simulink model "spm_control_sensorless_stc"  (R2021a)
settings: Solver=VariableStepAuto  StartTime=0.0  StopTime=3.0  FixedStep=1e-4  RelTol=1e-5
InitFcn:
  | bldc_data
  | test_data
values from neighbouring files (symbols this model uses):
  b = T_nom/Q_nom    (= 61.8430636014)    [bldc_data.m]
  current_limit = 300    [bldc_data.m]
  flux_obs_gain = 4e4    (= 40000)    [bldc_data.m]
  Jm = 0.3*0.05^2    (= 0.00075)    [bldc_data.m]
  theta_obs_gain = 2e6    (= 2000000)    [bldc_data.m]
undefined symbols (not defined in the file or in its folder): fluid, p, pmsm, r, speed_obs, stc
libraries: mcbcontrolslib x4, pid_lib x3, autolibpmsmexterior x1
settings Model: OrderedModelArguments=off  Creator=Rodrigo  LastModifiedBy=Rodrigo

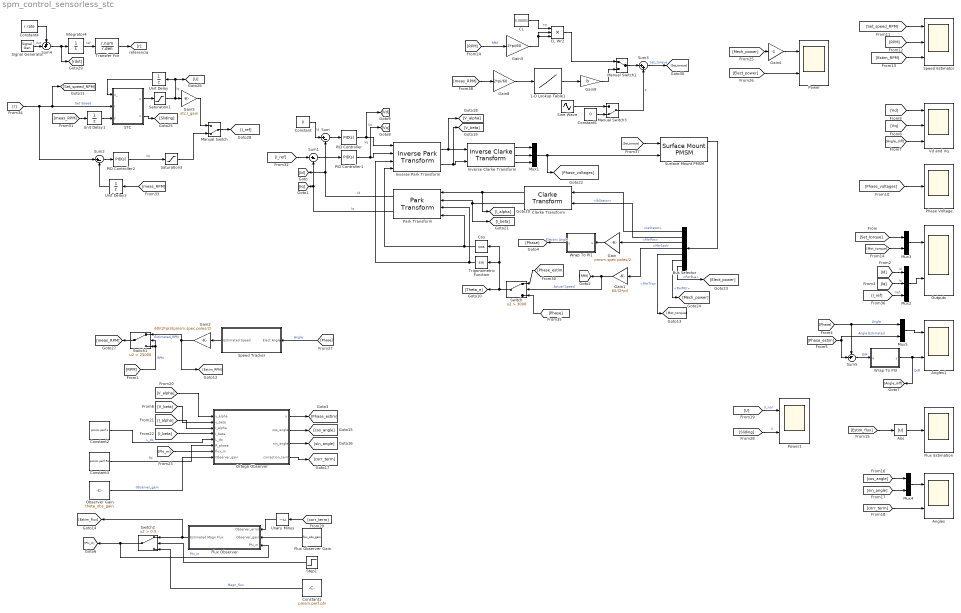
== system spm_control_sensorless_stc ==
  1-D Lookup Table1 : Lookup_n-D  NumberOfTableDimensions=1  BreakpointsForDimension1=fluid.W  Table=fluid.P  InternalRulePriority=Speed  RndMeth=Simplest  InputSameDT=on
  Abs : Abs
  Angles : Scope  NumInputPorts=2
  Angles1 : Scope  NumInputPorts=2
  Bus Selector : BusSelector  OutputSignals=IaStator,IbStator,MtrPos,MtrSpd,MtrTrq,PwrInfo.PwrTrnsfrd.PwrMtr,PwrInfo.PwrTrnsfrd.PwrBus
  CL : Constant  Value=0.00001
  CL Wr2 : Product  Inputs=3
  Clarke Transform : mcbcontrolslib/Clarke Transform  VariantControl=Variant2
  Constant : Constant  Value=0
  Constant1 : Constant  Value=pmsm.perf.phi
  Constant2 : Constant  Value=pmsm.perf.L
  Constant3 : Constant  Value=pmsm.perf.Rs
  Constant4 : Constant  Value=r.rate
  Constant5 : Constant  Value=0
  Cos : Trigonometry  Operator=cos
  Flux Estimation : Scope
  Flux Observer : Subsystem
  Flux Observer Gain : Constant  Value=flux_obs_gain
  Gain : Gain  Gain=pmsm.spec.poles/2
  Gain1 : Gain  Gain=60/(2*pi)
  Gain2 : Gain  Gain=60/(2*pi)/(pmsm.spec.poles/2)
  Gain3 : Gain  Gain=2*pi/60
  Gain4 : Gain  Gain=-1
  Gain5 : Gain  Gain=stc.I_gain
  Gain8 : Gain  Gain=2*pi/60
  Gain9 : Gain  Gain=b
  Integrator4 : Integrator  InitialCondition=r.off  LimitOutput=on  UpperSaturationLimit=r.lim  LowerSaturationLimit=0
  Inverse Clarke Transform : mcbcontrolslib/Inverse Clarke Transform
      settings: SourceProductBaseCode=MT
  Inverse Park Transform : mcbcontrolslib/Inverse Park Transform  AxisAlignment=D-axis
  Manual Switch : ManualSwitch  CurrentSetting=0
  Manual Switch1 : ManualSwitch
  Manual Switch3 : ManualSwitch  CurrentSetting=0
  Mux1 : Mux  Inputs=3
  Mux2 : Mux  Inputs=3
  Mux3 : Mux  Inputs=2
  Mux4 : Mux  Inputs=2
  Mux5 : Mux  Inputs=2
  Observer Gain : Constant  Value=theta_obs_gain
  Ortega Observer : Subsystem
  Outputs : Scope  NumInputPorts=2
  PID Controller : pid_lib/PID Controller  Controller=PID  Form=Parallel  TimeDomain=Continuous-time  UseExternalTs=off  SampleTime=-1  IntegratorMethod=Forward Euler  FilterMethod=Forward Euler  ControllerParametersSource=internal  P=3  I=0.3  D=0.1  UseFilter=on  N=100  TunerSelectOption=Transfer Function Based (PID Tuner App)  InitialConditionSource=internal  InitialConditionForIntegrator=0  InitialConditionForFilter=0  DifferentiatorICPrevScaledInput=0  ExternalReset=none  TrackingMode=off  Kt=1  LimitOutput=off  SatLimitsSource=internal  UpperSaturationLimit=inf  LowerSaturationLimit=-inf  LinearizeAsGain=on  AntiWindupMode=none  Kb=1  POutMin=[]  POutMax=[]  IOutMin=[]  IOutMax=[]  DOutMin=[]  DOutMax=[]  NOutMin=[]  NOutMax=[]  SumOutMin=[]  SumOutMax=[]  SaturationOutMin=[]  SaturationOutMax=[]  PParamMin=[]  PParamMax=[]  IParamMin=[]  IParamMax=[]  DParamMin=[]  DParamMax=[]  NParamMin=[]  NParamMax=[]  KbParamMin=[]  KbParamMax=[]  KtParamMin=[]  KtParamMax=[]  KbOutMin=[]  KbOutMax=[]  KtOutMin=[]  KtOutMax=[]  IntegratorOutMin=[]  IntegratorOutMax=[]  FilterOutMin=[]  FilterOutMax=[]  SumI1OutMin=[]  SumI1OutMax=[]  SumI2OutMin=[]  SumI2OutMax=[]  SumI3OutMin=[]  SumI3OutMax=[]  SumI4OutMin=[]  SumI4OutMax=[]  SumDOutMin=[]  SumDOutMax=[]  DifferentiatorOutMin=[]  DifferentiatorOutMax=[]  FilterDiffOutCoefMin=[]  FilterDiffOutCoefMax=[]  ReciprocalOutMin=[]  ReciprocalOutMax=[]  SumDenOutMin=[]  SumDenOutMax=[]  SumNumOutMin=[]  SumNumOutMax=[]  DivideOutMin=[]  DivideOutMax=[]  UdiffTsProdOutMin=[]  UdiffTsProdOutMax=[]  NTsProdOutMin=[]  NTsProdOutMax=[]  UintegralTsProdOutMin=[]  UintegralTsProdOutMax=[]  UngainTsProdOutMin=[]  UngainTsProdOutMax=[]  IntegratorContinuousStateAttributes=''  IntegratorStateMustResolveToSignalObject=off  IntegratorRTWStateStorageClass=Auto  FilterContinuousStateAttributes=''  FilterStateMustResolveToSignalObject=off  FilterRTWStateStorageClass=Auto  ParallelPVariant=InternalParameters  IdealPVariant=Disabled  IVariant=InternalParameters  DVariant=InternalParameters  IntegratorVariant=Continuous  SatVariant=Disabled  AWVariant=Passthrough  PCopyVariant=Disabled  TRVariant=Disabled  FdbkBlocksVariant=Forward  IdealPFdbkVariant=Disabled  SatFdbkVariant=Disabled  DerivativeFilterVariant=ContFilter  NVariant=InternalParameters  NCopyVariant=Disabled  FilterICVariant=InternalICsFilter  IntegratorICVariant=InternalICs  ExternalResetVariant=Disabled  TRSumVariant=Passthrough  SumFdbkVariant=Disabled  SumVariant=Sum_PID  TsampFilterVariant=InternalTs  TsampNgainVariant=Passthrough  TsampIntegralVariant=Passthrough  ExternalSaturationOutDataTypeStr=Inherit: Same as second input
  PID Controller1 : pid_lib/PID Controller  Controller=PID  Form=Parallel  TimeDomain=Continuous-time  UseExternalTs=off  SampleTime=-1  IntegratorMethod=Forward Euler  FilterMethod=Forward Euler  ControllerParametersSource=internal  P=6  I=2  D=0.3  UseFilter=on  N=100  TunerSelectOption=Transfer Function Based (PID Tuner App)  InitialConditionSource=internal  InitialConditionForIntegrator=0  InitialConditionForFilter=0  DifferentiatorICPrevScaledInput=0  ExternalReset=none  TrackingMode=off  Kt=1  LimitOutput=off  SatLimitsSource=internal  UpperSaturationLimit=inf  LowerSaturationLimit=-inf  LinearizeAsGain=on  AntiWindupMode=none  Kb=1  POutMin=[]  POutMax=[]  IOutMin=[]  IOutMax=[]  DOutMin=[]  DOutMax=[]  NOutMin=[]  NOutMax=[]  SumOutMin=[]  SumOutMax=[]  SaturationOutMin=[]  SaturationOutMax=[]  PParamMin=[]  PParamMax=[]  IParamMin=[]  IParamMax=[]  DParamMin=[]  DParamMax=[]  NParamMin=[]  NParamMax=[]  KbParamMin=[]  KbParamMax=[]  KtParamMin=[]  KtParamMax=[]  KbOutMin=[]  KbOutMax=[]  KtOutMin=[]  KtOutMax=[]  IntegratorOutMin=[]  IntegratorOutMax=[]  FilterOutMin=[]  FilterOutMax=[]  SumI1OutMin=[]  SumI1OutMax=[]  SumI2OutMin=[]  SumI2OutMax=[]  SumI3OutMin=[]  SumI3OutMax=[]  SumI4OutMin=[]  SumI4OutMax=[]  SumDOutMin=[]  SumDOutMax=[]  DifferentiatorOutMin=[]  DifferentiatorOutMax=[]  FilterDiffOutCoefMin=[]  FilterDiffOutCoefMax=[]  ReciprocalOutMin=[]  ReciprocalOutMax=[]  SumDenOutMin=[]  SumDenOutMax=[]  SumNumOutMin=[]  SumNumOutMax=[]  DivideOutMin=[]  DivideOutMax=[]  UdiffTsProdOutMin=[]  UdiffTsProdOutMax=[]  NTsProdOutMin=[]  NTsProdOutMax=[]  UintegralTsProdOutMin=[]  UintegralTsProdOutMax=[]  UngainTsProdOutMin=[]  UngainTsProdOutMax=[]  IntegratorContinuousStateAttributes=''  IntegratorStateMustResolveToSignalObject=off  IntegratorRTWStateStorageClass=Auto  FilterContinuousStateAttributes=''  FilterStateMustResolveToSignalObject=off  FilterRTWStateStorageClass=Auto  ParallelPVariant=InternalParameters  IdealPVariant=Disabled  IVariant=InternalParameters  DVariant=InternalParameters  IntegratorVariant=Continuous  SatVariant=Disabled  AWVariant=Passthrough  PCopyVariant=Disabled  TRVariant=Disabled  FdbkBlocksVariant=Forward  IdealPFdbkVariant=Disabled  SatFdbkVariant=Disabled  DerivativeFilterVariant=ContFilter  NVariant=InternalParameters  NCopyVariant=Disabled  FilterICVariant=InternalICsFilter  IntegratorICVariant=InternalICs  ExternalResetVariant=Disabled  TRSumVariant=Passthrough  SumFdbkVariant=Disabled  SumVariant=Sum_PID  TsampFilterVariant=InternalTs  TsampNgainVariant=Passthrough  TsampIntegralVariant=Passthrough  ExternalSaturationOutDataTypeStr=Inherit: Same as second input
  PID Controller2 : pid_lib/PID Controller  Controller=PID  Form=Parallel  TimeDomain=Continuous-time  UseExternalTs=off  SampleTime=-1  IntegratorMethod=Forward Euler  FilterMethod=Forward Euler  ControllerParametersSource=internal  P=0.009  I=0.06  D=0  UseFilter=on  N=100  TunerSelectOption=Transfer Function Based (PID Tuner App)  InitialConditionSource=internal  InitialConditionForIntegrator=0  InitialConditionForFilter=0  DifferentiatorICPrevScaledInput=0  ExternalReset=none  TrackingMode=off  Kt=1  LimitOutput=off  SatLimitsSource=internal  UpperSaturationLimit=inf  LowerSaturationLimit=-inf  LinearizeAsGain=on  AntiWindupMode=none  Kb=1  POutMin=[]  POutMax=[]  IOutMin=[]  IOutMax=[]  DOutMin=[]  DOutMax=[]  NOutMin=[]  NOutMax=[]  SumOutMin=[]  SumOutMax=[]  SaturationOutMin=[]  SaturationOutMax=[]  PParamMin=[]  PParamMax=[]  IParamMin=[]  IParamMax=[]  DParamMin=[]  DParamMax=[]  NParamMin=[]  NParamMax=[]  KbParamMin=[]  KbParamMax=[]  KtParamMin=[]  KtParamMax=[]  KbOutMin=[]  KbOutMax=[]  KtOutMin=[]  KtOutMax=[]  IntegratorOutMin=[]  IntegratorOutMax=[]  FilterOutMin=[]  FilterOutMax=[]  SumI1OutMin=[]  SumI1OutMax=[]  SumI2OutMin=[]  SumI2OutMax=[]  SumI3OutMin=[]  SumI3OutMax=[]  SumI4OutMin=[]  SumI4OutMax=[]  SumDOutMin=[]  SumDOutMax=[]  DifferentiatorOutMin=[]  DifferentiatorOutMax=[]  FilterDiffOutCoefMin=[]  FilterDiffOutCoefMax=[]  ReciprocalOutMin=[]  ReciprocalOutMax=[]  SumDenOutMin=[]  SumDenOutMax=[]  SumNumOutMin=[]  SumNumOutMax=[]  DivideOutMin=[]  DivideOutMax=[]  UdiffTsProdOutMin=[]  UdiffTsProdOutMax=[]  NTsProdOutMin=[]  NTsProdOutMax=[]  UintegralTsProdOutMin=[]  UintegralTsProdOutMax=[]  UngainTsProdOutMin=[]  UngainTsProdOutMax=[]  IntegratorContinuousStateAttributes=''  IntegratorStateMustResolveToSignalObject=off  IntegratorRTWStateStorageClass=Auto  FilterContinuousStateAttributes=''  FilterStateMustResolveToSignalObject=off  FilterRTWStateStorageClass=Auto  ParallelPVariant=InternalParameters  IdealPVariant=Disabled  IVariant=InternalParameters  DVariant=InternalParameters  IntegratorVariant=Continuous  SatVariant=Disabled  AWVariant=Passthrough  PCopyVariant=Disabled  TRVariant=Disabled  FdbkBlocksVariant=Forward  IdealPFdbkVariant=Disabled  SatFdbkVariant=Disabled  DerivativeFilterVariant=ContFilter  NVariant=InternalParameters  NCopyVariant=Disabled  FilterICVariant=InternalICsFilter  IntegratorICVariant=InternalICs  ExternalResetVariant=Disabled  TRSumVariant=Passthrough  SumFdbkVariant=Disabled  SumVariant=Sum_PID  TsampFilterVariant=InternalTs  TsampNgainVariant=Passthrough  TsampIntegralVariant=Passthrough  ExternalSaturationOutDataTypeStr=Inherit: Same as second input
  Park Transform : mcbcontrolslib/Park Transform  AxisAlignment=D-axis
      settings: SourceProductBaseCode=MT
  Phase Voltage : Scope
  Power : Scope  NumInputPorts=2
  Power1 : Scope  NumInputPorts=2
  STC : MATLAB Function  TreatAsAtomicUnit=on  SystemSampleTime=stc.ts
  Saturation1 : Saturate  UpperLimit=stc.UM  LowerLimit=-stc.UM
  Saturation3 : Saturate  UpperLimit=current_limit  LowerLimit=-current_limit
  Signal Generator : SignalGenerator  Amplitude=r.a  Frequency=r.f
  Sine Wave : Sin  Amplitude=p.a  Frequency=p.w  SampleTime=0
  Speed Estimator : Scope  NumInputPorts=3
  Speed Tracker : Subsystem
  Step1 : Step  Time=0.01  After=2  SampleTime=0
  Sum : Sum  Inputs=|+-
  Sum1 : Sum  Inputs=|+-
  Sum2 : Sum  Inputs=|+-
  Sum3 : Sum  Inputs=|++
  Sum4 : Sum  Inputs=++|
  Sum5 : Sum  Inputs=-+|
  Surface Mount PMSM : autolibpmsmexterior/Surface Mount PMSM  port_config=Torque  sim_type=Continuous  Ts=0.001  P=pmsm.spec.poles/2  Rs=pmsm.perf.Rph  Ldq_=pmsm.perf.L  KConstText=Permanent flux linkage constant (lambda_pm):  lambda_pm=pmsm.perf.phi  Ke=159.9771  Kt=1.323  mechanical=[Jm, 0.0001, 0.2]  idq0=[0 0]  theta_init=0  omega_init=0  KConst=pmsm.perf.phi  lambda_pm_calc=pmsm.perf.phi  RefBlkName='autolibpmsmexterior/Surface Mount PMSM'  aMode=5  Ldq="[0.0017      0.0017]"
      settings: SourceProductBaseCode=PW,DR,MT,UV,VE
  Switch : Switch  Criteria=u2 > Threshold  Threshold=3000
  Switch1 : Switch  Criteria=u2 > Threshold  Threshold=25000
  Switch2 : Switch  Criteria=u2 > Threshold  Threshold=0.5
  Transfer Fcn : TransferFcn  Numerator=r.num  Denominator=r.den
  Trigonometric Function : Trigonometry
  Unary Minus : UnaryMinus
  Unit Delay : UnitDelay  SampleTime=-1  HasFrameUpgradeWarning=on
  Unit Delay1 : UnitDelay  SampleTime=-1  HasFrameUpgradeWarning=on
  Unit Delay2 : UnitDelay  SampleTime=-1  HasFrameUpgradeWarning=on
  Vd and Vq : Scope  NumInputPorts=3
  Wrap To PI1 : MATLAB Function  TreatAsAtomicUnit=on
  Wrap To PI3 : MATLAB Function  TreatAsAtomicUnit=on
  wires:
  Inverse Clarke Transform/1 -> Mux1/1
  Inverse Clarke Transform/2 -> Mux1/2
  Inverse Clarke Transform/3 -> Mux1/3
  Inverse Park Transform/1 -> [V_alpha], Inverse Clarke Transform/1
  Inverse Park Transform/2 -> [V_beta], Inverse Clarke Transform/2
  Clarke Transform/1 -> [I_alpha], Park Transform/1
  Clarke Transform/2 -> [I_beta], Park Transform/2
  PID Controller/1 -> [Vd], Inverse Park Transform/1  "Vd"
  PID Controller1/1 -> [Vq], Inverse Park Transform/2  "Vq"
  Sum/1 -> PID Controller/1
  Sum1/1 -> PID Controller1/1
  Park Transform/1 -> [Id], Sum/2  "Id"
  Park Transform/2 -> [Iq], Sum1/2  "Iq"
  Saturation1/1 -> Gain5/1, [U], Unit Delay/1  "Iq"
  Constant/1 -> Sum/1  "Id"
  Cos/1 -> Park Transform/4, Inverse Park Transform/4
  Trigonometric Function/1 -> Park Transform/3, Inverse Park Transform/3
  Surface Mount PMSM/1 -> Bus Selector/1
  Bus Selector/3 -> Gain/1  "<MtrPos>"
  Bus Selector/1 -> Clarke Transform/1  "<IaStator>"
  Bus Selector/2 -> Clarke Transform/2  "<IbStator>"
  Bus Selector/4 -> Gain1/1  "<MtrSpd>"
  [r] -> Sum2/1, [Set_speed_RPM], STC/2(r)  "Set Speed"
  Speed Tracker/1(Estimated Speed) -> Gain2/1
  Gain/1 -> Wrap To PI1/1(u)
  Wrap To PI1/1(y) -> [Phase]  "Electric Angle"
  Switch/1 -> Cos/1, Trigonometric Function/1, [Theta_e]
  Gain2/1 -> [Estim_RPM], Switch1/1  "Estimated_RPM"
  Gain1/1 -> Switch/2, [RPM]  "Actual Speed"
  [RPM] -> Switch1/2, Switch1/3  "RPM"
  [Set_torque] -> Mux3/1
  [Iq] -> Mux2/2  "Iq"
  [Id] -> Mux2/1  "Id"
  [Phase_estim] -> Sum5/2, Mux5/2  "Angle Estimated"
  [Phase] -> Mux5/1, Sum5/1  "Angle"
  Sum5/1 -> Wrap To PI3/1(u)  "Diff"
  Wrap To PI3/1(y) -> [Angle_diff], Angles1/2  "Diff"
  Mux3/1 -> Outputs/1
  Mux2/1 -> Outputs/2
  Mux4/1 -> Angles/1
  Mux5/1 -> Angles1/1
  [Angle_diff] -> Vd and Vq/3
  [Vd] -> Vd and Vq/1
  [Vq] -> Vd and Vq/2
  [Phase_voltages] -> Phase Voltage/1
  [Set_speed_RPM] -> Speed Estimator/1
  [RPM] -> Speed Estimator/2
  [Estim_RPM] -> Speed Estimator/3
  [Mot_torque] -> Mux3/2
  Bus Selector/5 -> [Mot_torque]  "<MtrTrq>"
  [cos_angle] -> Mux4/1
  [sin_angle] -> Mux4/2
  [corr_term] -> Angles/2
  [Estim_flux] -> Abs/1
  Abs/1 -> Flux Estimation/1
  Mux1/1 -> Surface Mount PMSM/2, [Phase_voltages]
  Bus Selector/6 -> [Mech_power]  "<PwrMtr>"
  Bus Selector/7 -> [Elect_power]  "<PwrBus>"
  [Elect_power] -> Power/2
  [Mech_power] -> Gain4/1
  Gain4/1 -> Power/1
  [Phase] -> Speed Tracker/1(Elect Angle)  "Angle"
  Unit Delay/1 -> STC/1(u_)
  STC/1(u) -> Saturation1/1
  STC/2(s) -> [Sliding]
  [U] -> Power1/1  "U_nor"
  [Sliding] -> Power1/2  "S"
  [RPM] -> Gain3/1  "RPM"
  CL/1 -> CL Wr2/1  "T0"
  Gain3/1 -> CL Wr2/3, CL Wr2/2
  CL Wr2/1 -> Manual Switch1/1
  Unit Delay1/1 -> STC/3(y)
  Switch1/1 -> [meas_RPM]
  [meas_RPM] -> Unit Delay1/1
  [I_ref] -> Sum1/1
  Sum2/1 -> PID Controller2/1
  Manual Switch/1 -> [I_ref]
  Gain5/1 -> Manual Switch/1
  PID Controller2/1 -> Saturation3/1  "Vq"
  Sum4/1 -> [rdot], Integrator4/1
  Signal Generator/1 -> Sum4/2  "r_dot"
  Constant4/1 -> Sum4/1
  Transfer Fcn/1 -> [r]
  Integrator4/1 -> Transfer Fcn/1  "ref"
  Constant5/1 -> Manual Switch3/2
  Manual Switch3/1 -> Sum3/2  "p"
  Sine Wave/1 -> Manual Switch3/1
  [Set_torque] -> Surface Mount PMSM/1
  Gain8/1 -> 1-D Lookup Table1/1
  [meas_RPM] -> Gain8/1
  1-D Lookup Table1/1 -> Gain9/1
  Manual Switch1/1 -> Sum3/1
  Gain9/1 -> Manual Switch1/2
  Sum3/1 -> [Set_torque]  "Set_torque"
  Switch2/1 -> Flux Observer/3(Phi_m), [Phi_m]  "Phi_m"
  Ortega Observer/2(cos_angle) -> [cos_angle]
  Step1/1 -> Switch2/2
  Unary Minus/1 -> Flux Observer/1(Observer_error)
  [Phi_m] -> Ortega Observer/7(flux_m)
  Constant3/1 -> Ortega Observer/6(R_phase)  "Rs"
  [corr_term] -> Unary Minus/1
  Constant2/1 -> Ortega Observer/5(L_dq)  "L_dq"
  [V_beta] -> Ortega Observer/2(v_beta)
  Ortega Observer/4(correction_term) -> [corr_term]
  [V_alpha] -> Ortega Observer/1(v_alpha)
  [I_beta] -> Ortega Observer/4(i_beta)
  [I_alpha] -> Ortega Observer/3(i_alpha)
  Ortega Observer/3(sin_angle) -> [sin_angle]
  Flux Observer/1(Estimated Magn Flux) -> [Estim_flux], Switch2/1
  Flux Observer Gain/1 -> Flux Observer/2(Observer_gain)
  Observer Gain/1 -> Ortega Observer/8(Observer_gain)  "Observer_gain"
  Ortega Observer/1(y) -> [Phase_estim]
  Constant1/1 -> Switch2/3  "Magn_flux"
  [Phase] -> Switch/3
  [Phase_estim] -> Switch/1
  [meas_RPM] -> Unit Delay2/1
  Unit Delay2/1 -> Sum2/2
  [I_ref] -> Mux2/3  "Iref"
  Saturation3/1 -> Manual Switch/2

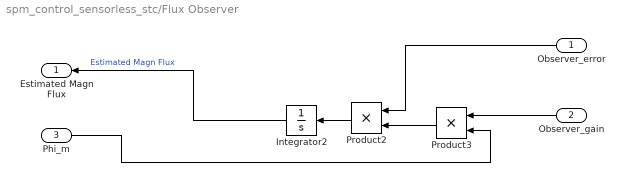
== system spm_control_sensorless_stc/Flux Observer ==
  Observer_error : Inport
  Observer_gain : Inport  Port=2
  Phi_m : Inport  Port=3
  Integrator2 : Integrator
  Product2 : Product
  Product3 : Product
  Estimated Magn Flux : Outport
  wires:
  Product3/1 -> Product2/2
  Product2/1 -> Integrator2/1
  Observer_error/1 -> Product2/1
  Observer_gain/1 -> Product3/1
  Phi_m/1 -> Product3/2
  Integrator2/1 -> Estimated Magn Flux/1  "Estimated Magn Flux"

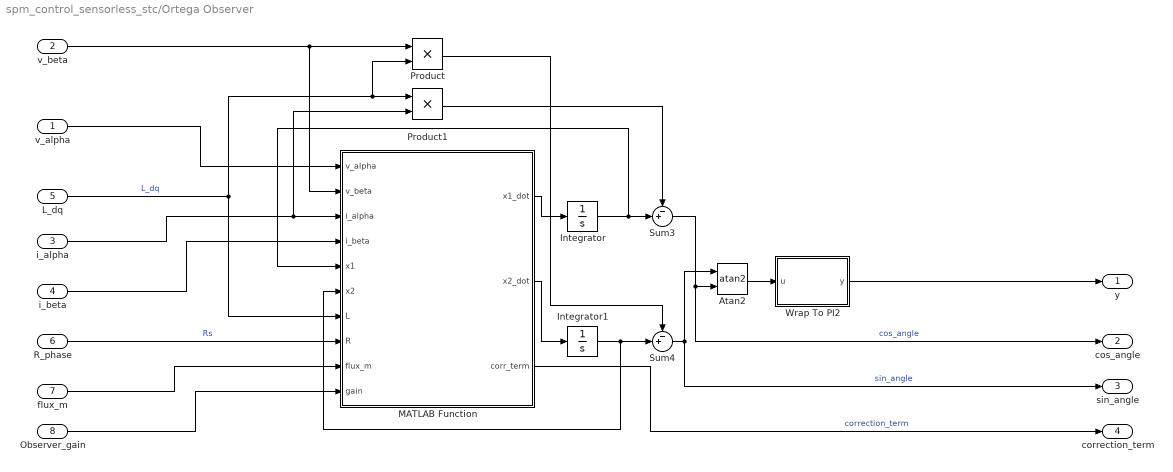
== system spm_control_sensorless_stc/Ortega Observer ==
  v_alpha : Inport
  v_beta : Inport  Port=2
  i_alpha : Inport  Port=3
  i_beta : Inport  Port=4
  L_dq : Inport  Port=5
  R_phase : Inport  Port=6
  flux_m : Inport  Port=7
  Observer_gain : Inport  Port=8
  Atan2 : Trigonometry  Operator=atan2
  Integrator : Integrator
  Integrator1 : Integrator
  MATLAB Function : MATLAB Function  TreatAsAtomicUnit=on
  Product : Product
  Product1 : Product
  Sum3 : Sum  Inputs=-+|
  Sum4 : Sum  Inputs=-+|
  Wrap To PI2 : MATLAB Function  TreatAsAtomicUnit=on
  y : Outport
  cos_angle : Outport  Port=2
  sin_angle : Outport  Port=3
  correction_term : Outport  Port=4
  wires:
  i_alpha/1 -> MATLAB Function/3(i_alpha), Product1/2
  L_dq/1 -> MATLAB Function/7(L), Product/2, Product1/1  "L_dq"
  Integrator1/1 -> Sum4/2, MATLAB Function/6(x2)
  MATLAB Function/1(x1_dot) -> Integrator/1
  v_beta/1 -> MATLAB Function/2(v_beta), Product/1
  Atan2/1 -> Wrap To PI2/1(u)
  Product/1 -> Sum4/1
  Wrap To PI2/1(y) -> y/1
  Integrator/1 -> Sum3/2, MATLAB Function/5(x1)
  Sum4/1 -> sin_angle/1, Atan2/1  "sin_angle"
  Sum3/1 -> cos_angle/1, Atan2/2  "cos_angle"
  Product1/1 -> Sum3/1
  MATLAB Function/3(corr_term) -> correction_term/1  "correction_term"
  flux_m/1 -> MATLAB Function/9(flux_m)
  Observer_gain/1 -> MATLAB Function/10(gain)
  R_phase/1 -> MATLAB Function/8(R)  "Rs"
  MATLAB Function/2(x2_dot) -> Integrator1/1
  i_beta/1 -> MATLAB Function/4(i_beta)
  v_alpha/1 -> MATLAB Function/1(v_alpha)

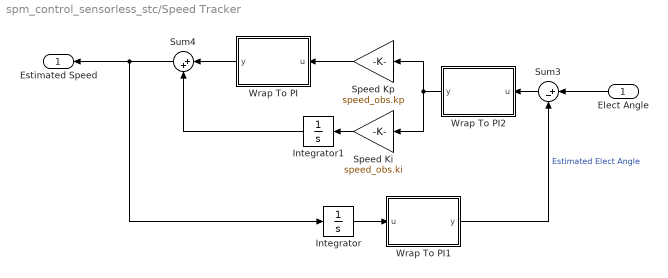
== system spm_control_sensorless_stc/Speed Tracker ==
  Elect Angle : Inport
  Integrator : Integrator
  Integrator1 : Integrator
  Speed Ki : Gain  Gain=speed_obs.ki
  Speed Kp : Gain  Gain=speed_obs.kp
  Sum3 : Sum  Inputs=|+-
  Sum4 : Sum  Inputs=|++
  Wrap To PI : MATLAB Function  TreatAsAtomicUnit=on
  Wrap To PI1 : MATLAB Function  TreatAsAtomicUnit=on
  Wrap To PI2 : MATLAB Function  TreatAsAtomicUnit=on
  Estimated Speed : Outport
  wires:
  Speed Ki/1 -> Integrator1/1
  Integrator1/1 -> Sum4/2
  Sum4/1 -> Estimated Speed/1, Integrator/1
  Integrator/1 -> Wrap To PI1/1(u)
  Wrap To PI/1(y) -> Sum4/1
  Speed Kp/1 -> Wrap To PI/1(u)
  Wrap To PI1/1(y) -> Sum3/2  "Estimated Elect Angle"
  Elect Angle/1 -> Sum3/1
  Sum3/1 -> Wrap To PI2/1(u)
  Wrap To PI2/1(y) -> Speed Kp/1, Speed Ki/1

== matlab function spm_control_sensorless_stc/Speed Tracker/Wrap To PI1 ==
  data: u input; y output
function y = fcn(u)

y = wrapToPi(u);

== matlab function spm_control_sensorless_stc/Speed Tracker/Wrap To PI ==
  data: u input; y output
function y = fcn(u)

y = wrapToPi(u);

== matlab function spm_control_sensorless_stc/Ortega Observer/MATLAB Function ==
  data: v_alpha input; x1_dot output; v_beta input; i_alpha input; i_beta input; x2_dot output; x1 input; x2 input; L input; R input; flux_m input; gain input; corr_term output
function [x1_dot,x2_dot,corr_term] = ortega_obs(v_alpha, v_beta, i_alpha, i_beta, x1, x2, L, R, flux_m, gain)

corr_term = flux_m^2 - ((x1 - L*i_alpha)^2 + (x2 - L*i_beta)^2);

% if(corr_term < 0)
%      corr_term = 0;
% end

x1_dot = v_alpha - R*i_alpha + gain/2 * (x1 - L*i_alpha) * corr_term;
x2_dot = v_beta - R*i_beta + gain/2 * (x2 - L*i_beta) * corr_term;

== matlab function spm_control_sensorless_stc/Wrap To PI1 ==
  data: u input; y output
function y = fcn(u)

y = wrapToPi(u);

== matlab function spm_control_sensorless_stc/Ortega Observer/Wrap To PI2 ==
  data: u input; y output
function y = fcn(u)

y = wrapToPi(u);

== matlab function spm_control_sensorless_stc/Speed Tracker/Wrap To PI2 ==
  data: u input; y output
function y = fcn(u)

y = wrapToPi(u);

== matlab function spm_control_sensorless_stc/Wrap To PI3 ==
  data: u input; y output
function y = fcn(u)

y = wrapToPi(u);

== matlab function spm_control_sensorless_stc/STC ==
  data: u_ input size=1; r input size=1; y input size=1; u output size=1; s output size=1; stc parameter size=1
% r : referencia
% y : medicion
% u_: accion de control precedente
% stc: configuracion (cargada en el workspace) con campos 
%      .l1 : ganancia proporcional
%      .l2 : ganancia integral
%      .ts : tiempo de muestreo

function [u, s] = pos_dstc(u_, r, y, stc) 
    persistent up % componente proporcional
    if isempty(up)
        up = 0;
    end
    s  = y - r;   % variable de deslizamiento
    ui = u_ - up;     
    [up, ui] = dstc_imp(ui, s, stc.l1, stc.l2, stc.ts);
    u = up + ui;  % accion de control
end 

% up: parte proporcional
% ui: parte integral
function [up, ui] = dstc_imp(ui, s, l1, l2, ts) 
    a    = ts* l1;
    hl2  = ts* l2;
    h2l2 = hl2 * ts;
    bk = -s - ts*ui;
    if     bk <-h2l2
        z  = (sqrt(a^2 - 4*(bk + h2l2))-a)/2;
        ui =  ui - hl2;
        up = -l1*z;
    elseif bk > h2l2
        z  = (sqrt(a^2 + 4*(bk - h2l2))-a)/2;
        ui =  ui + hl2;
        up =  l1*z;
    else
        ui = -s / ts;
        up =  0;
    end
end
